simulink model "HEMS_leon"  (R2023b)
settings: Solver=FixedStepDiscrete  StartTime=0.0  StopTime=T_end  FixedStep=Ts  RelTol=1e-3  EnableMultiTasking=on
InitFcn:
  | % stepsize is now 1 per seconds cause 1 step is 1 minute
  | 
  | Ts=1/60;% 1Ts = 1minute => 60TimeSteps = 1hour
  | 
  | % Simulation Time
  | T_end = 24; % = 24 hours
StopFcn:
  | %
values from neighbouring files (symbols this model uses):
  battery_capacity = 15    [RBC.m]    (also in plot_results_HEMS.m = evalin('base', 'battery_capacity'))
  battery_efficiency = 0.95    [RBC.m]
  battery_max_charge = 5    [RBC.m]
  battery_max_soc = 90    [RBC.m]    (also in plot_results_HEMS.m = evalin('base', 'battery_max_soc'))
  battery_min_soc = 20    [RBC.m]    (also in plot_results_HEMS.m = evalin('base', 'battery_min_soc'))
  battery_soc_initial = 40    [RBC.m]
undefined symbols (not defined in the file or in its folder): A, B, battEnergy, C, D, DiscIntNeverNeededParam, optTime, x0
libraries: dspsigops x1, spspowerguiLib x1
settings Model: Creator=mas  LastModifiedBy=leons
settings SolverCC: AlgebraicLoopSolver=TrustRegion  AutoInsertRateTranBlk=on
settings DataIOCC: LimitDataPoints=on  SaveFormat=Array  SignalLoggingSaveFormat=ModelDataLogs  SaveTime=off  ReturnWorkspaceOutputs=off
settings OptimizationCC: ExpressionDepthLimit=2147483647  LifeSpan=inf
settings DebuggingCC: UnderspecifiedInitializationDetection=Classic  MergeDetectMultiDrivingBlocksExec=none  SolverPrmCheckMsg=warning  FcnCallInpInsideContextMsg=warning  UnconnectedInputMsg=warning  UnconnectedOutputMsg=warning  UnconnectedLineMsg=warning  StateNameClashWarn=warning  SFUnexpectedBacktrackingDiag=warning  SFNoUnconditionalDefaultTransitionDiag=warning  SFExecutionAtInitializationDiag=none  ArithmeticOperatorsInVariantConditions=warning
settings HardwareCC: ProdBitPerPointer=32  ProdBitPerSizeT=32  ProdBitPerPtrDiffT=32  ProdLargestAtomicFloat=None  ProdIntDivRoundTo=Undefined  ProdEndianess=Unspecified  ProdWordSize=32  ProdHWDeviceType=32-bit Generic
settings ModelReferenceCC: EnableRefExpFcnMdlSchedulingChecks=on  PropagateSignalLabelsOutOfModel=off
settings SFSimCC: SimUseLocalCustomCode=off  CustomCodeUndefinedFunction=UseInterfaceOnly
settings RTWCC: RTWUseLocalCustomCode=off  DLArmComputeVersion=19.05
settings CodeAppCC: StateflowObjectComments=on
settings GRTTargetCC: TargetLangStandard=C89/C90 (ANSI)  CombineOutputUpdateFcns=off  GRTInterface=on
settings ConfigComp: CovMetricSettings=dw  CovSaveCumulativeToWorkspaceVar=on  CovSaveSingleToWorkspaceVar=on  CovExternalEMLEnable=off  CovSFcnEnable=off

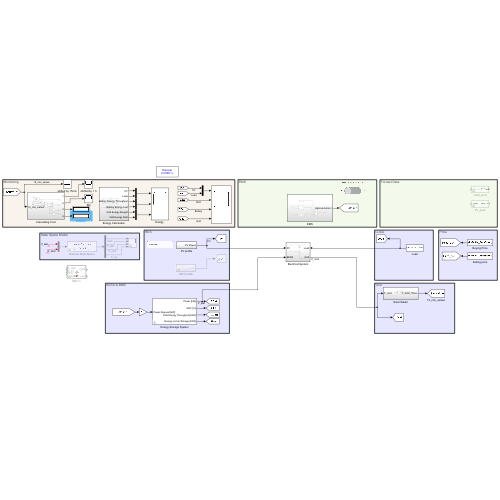
[thumbnail: Simulink's stored preview of the top-level diagram]
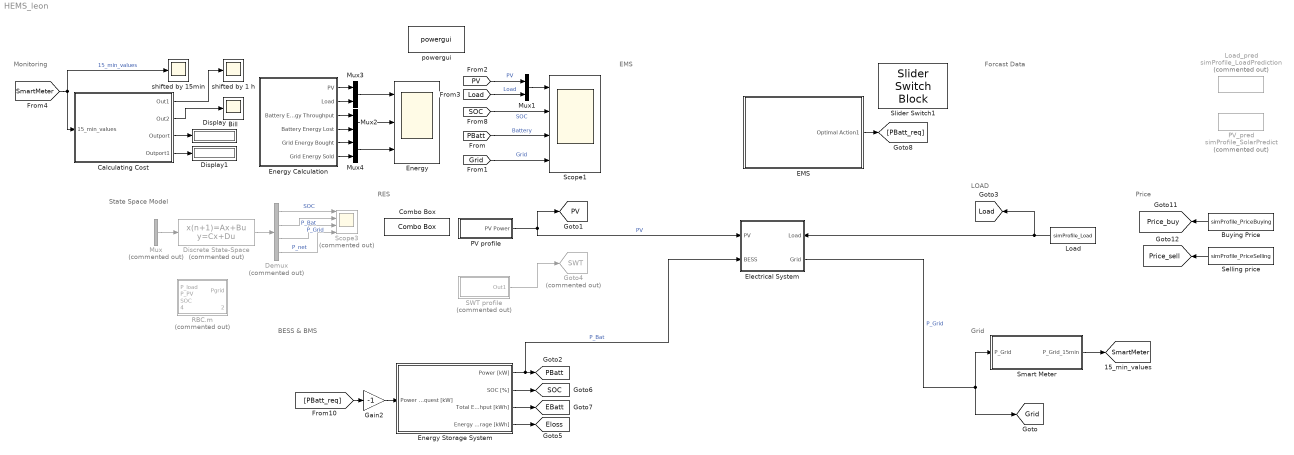
== system HEMS_leon ==
  note: State Space Model
  note: Grid
  note: BESS & BMS
  note: RES
  note: LOAD
  note: EMS
  note: Monitoring
  note: Forcast Data
  note: Price
  Bill : Scope
  Buying Price : FromWorkspace  VariableName=simProfile_PriceBuying  SampleTime=Ts*60  Interpolate=off  OutputAfterFinalValue=Holding final value
  Calculating Cost : Subsystem
  Combo Box : ComboBox  LabelPosition=Hide  SelectedLabel=Cloudy Day
      settings: Values={{'Cloudy Day', 'ClearDay'}, [1 0]}
  Demux : Demux  Commented=on
  Discrete State-Space : DiscreteStateSpace  Commented=on  A=A  B=B  C=C  D=D  InitialCondition=x0  SampleTime=-1
  Display : Display
  Display1 : Display
  EMS : Subsystem
  Electrical System : Subsystem
      settings: PortSchema="{\"entries\":[{\"content\":{\"sides\":[{\"content\":{\"connectorIds\":[\"In1\",\"Out1\"]},\"type\":\"ConnectorPlacement.EquallySpacedRectSide\",\"uuid\":\"ea2d6f6f-0b16-4ab1-9278-b701b85b7cf6\"},{\"content\":{\"connectorIds\":[\"In2\",\"In3\"],\"side\":\"RIGHT\"},\"type\":\"ConnectorPlacement.EquallySpacedRectSide\",\"uuid\":\"7f792676-012d-49e4-aa54-4a4cf568511b\"},{\"content\":{\"side\":\"TOP\"},\"type\":\"ConnectorPlacement.EquallySpacedRectSide\",\"uuid\":\"0f596cfa-1807-49b9-975a-a3b3036f9244\"}]},\"type\":\"ConnectorPlacement.EquallySpacedConnector\",\"uuid\":\"02bb58de-c0fd-4021-befc-2f3cc3c5a74e\"}],\"packageUris\":[\"http://schema.mathworks.com/mf0/Connector/R2020b\"],\"version\":\"1.0\"}"
  "Energy " : Scope  NumInputPorts=3
  Energy Calculation : Subsystem
  Energy Storage System : Subsystem  mask{Pmax=battery_max_charge, Emax=battery_capacity, SOCinit=battery_soc_initial, Eff=battery_efficiency*100, SOCmax=battery_max_soc, SOCmin=battery_min_soc}
      mask prompts: Pmax "Max Power [kW] (both for charging and discharging)"; Emax "Total Storage Energy [kWh]"; SOCinit "Initial SOC [%]"; Eff "Round Trip Efficiency [%]"; SOCmax "SOC max"; SOCmin "SOC min"
  Gain2 : Gain  Gain=-1
  Goto4 : Goto  Commented=on  GotoTag=SWT  TagVisibility=global
  Load : FromWorkspace  VariableName=simProfile_Load  SampleTime=Ts  OutputAfterFinalValue=Holding final value
  Load_pred : FromWorkspace  Commented=on  VariableName=simProfile_LoadPrediction  SampleTime=Ts  OutputAfterFinalValue=Holding final value
  Mux : Mux  Commented=on  Inputs=2
  Mux{1..4} (4 alike) : Mux  Inputs=2
  PV profile : Subsystem
  PV_pred : FromWorkspace  Commented=on  VariableName=simProfile_SolarPredict  SampleTime=Ts  OutputAfterFinalValue=Holding final value
  RBC.m : MATLAB Function  Commented=on  TreatAsAtomicUnit=on
  SWT profile : Subsystem  Commented=on
  Scope1 : Scope  NumInputPorts=4
  Scope3 : Scope  Commented=on  NumInputPorts=4
  Selling price : FromWorkspace  VariableName=simProfile_PriceSelling  SampleTime=Ts*60  Interpolate=off  OutputAfterFinalValue=Holding final value
  Slider Switch1 : SliderSwitchBlock
      settings: Values={{'RBC', 'OPT'}, [0 1]}
  Smart Meter : Subsystem
  powergui : spspowerguiLib/powergui  Priority=1  SimulationMode=Discrete  SampleTime=Ts  frequency=60  Iterations=50  frequencyindice=60  Pbase=100e6  ErrMax=1e-4  UnitsV=kV  UnitsW=MW  buscounter=0  FunctionMessages=off  echomessages=off  EnableUseOfTLC=off  CurrentSourceSwitches=off  DisableSnubberDevices=off  DisableRonSwitches=off  DisableVfSwitches=off  DisplayEquations=off  AutomaticDiscreteSolvers=off  SolverType=Tustin/Backward Euler (TBE)  Interpol=off  ExternalGateDelay=off  methode=off  Ts=100  x0status=blocks  SPID=on  SwTol=0  HookPort=off  NonlinearTolerance=1e-4  nMaxIteration=100  ContinueOnMaxIteration=off  RestoreLinks=warning  ResistiveCurrentMeasurement=off  Frange=[0:2:500]  Ylog=off  Xlog=on  ShowGrid=off  save=off  variable=ZData  structure=0  ZoomFFT=off  StartTime=0.0  cycles=1  DisplayStyle=1  fundamental=60  FreqAxis=off  MaxFrequency=1000  frequencyindicesteady=1  RmsSteady=1  display=off
  shifted by 1 h : Scope
  shifted by 15min : Scope
  tag scope: EBatt=global, Eloss=global, Grid=global, Load=global, PBatt=global, PV=global, Price_buy=global, Price_sell=global, SOC=global, SmartMeter=global
  wires:
  Energy Storage System/2(SOC [%]) -> [SOC]
  Energy Storage System/3(Total Energy Throughput [kWh]) -> [EBatt]
  PV profile/1(PV Power) -> [PV], Electrical System/2(PV)  "PV"
  Gain2/1 -> Energy Storage System/1(Power Request [kW])
  [Load] -> Mux1/2  "Load"
  [PBatt] -> Scope1/3  "Battery"
  [PV] -> Mux1/1  "PV"
  [Grid] -> Scope1/4  "Grid"
  Mux2/1 -> "Energy "/2
  Energy Storage System/4(" Energy Lost in Storage [kWh]") -> [Eloss]
  Energy Storage System/1(Power [kW]) -> Electrical System/3(BESS), [PBatt]  "P_Bat"
  Electrical System/1(Grid) -> Smart Meter/1(P_Grid), [Grid]  "P_Grid"
  Load/1 -> Electrical System/1(Load), [Load]
  ? -> Mux/2  "P_Grid"
  Demux/2 -> Scope3/2  "P_Bat"
  Demux/4 -> Scope3/4  "P_net"
  Mux/1 -> Discrete State-Space/1
  ? -> Mux/1  "P_Bat"
  Discrete State-Space/1 -> Demux/1
  Demux/1 -> Scope3/1  "SOC"
  Demux/3 -> Scope3/3  "P_Grid"
  Mux1/1 -> Scope1/1
  [SOC] -> Scope1/2  "SOC"
  Mux3/1 -> "Energy "/1
  Mux4/1 -> "Energy "/3
  EMS/1(Optimal Action1) -> [PBatt_req]
  [PBatt_req] -> Gain2/1
  Energy Calculation/1(PV) -> Mux3/1
  Energy Calculation/2(Load) -> Mux3/2
  Energy Calculation/3(Battery Energy Throughput) -> Mux2/1
  Energy Calculation/4(Battery Energy Lost) -> Mux2/2
  Energy Calculation/5(Grid Energy Bought) -> Mux4/1
  Energy Calculation/6(Grid Energy Sold) -> Mux4/2
  [SmartMeter] -> shifted by 15min/1, Calculating Cost/1(15_min_values)  "15_min_values"
  Buying Price/1 -> [Price_buy]
  Selling price/1 -> [Price_sell]
  Calculating Cost/1(Out1) -> shifted by 1 h/1
  Calculating Cost/2(Out2) -> Bill/1
  SWT profile/1(Out1) -> Goto4/1
  Smart Meter/1(P_Grid_15min) -> [SmartMeter]
  Calculating Cost/3(Outport) -> Display/1
  Calculating Cost/4(Outport1) -> Display1/1

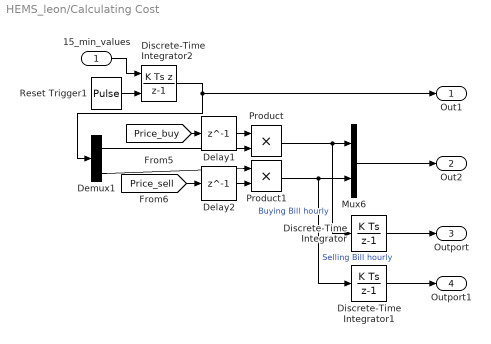
== system HEMS_leon/Calculating Cost ==
  15_min_values : Inport
  Delay1 : Delay  DelayLength=1
  Delay2 : Delay  DelayLength=1
  Demux1 : Demux  Outputs=2
  Discrete-Time Integrator : DiscreteIntegrator  SampleTime=-1  ICPrevOutput=DiscIntNeverNeededParam  ICPrevScaledInput=DiscIntNeverNeededParam
  Discrete-Time Integrator1 : DiscreteIntegrator  SampleTime=-1  ICPrevOutput=DiscIntNeverNeededParam  ICPrevScaledInput=DiscIntNeverNeededParam
  Discrete-Time Integrator2 : DiscreteIntegrator  IntegratorMethod=Integration: Backward Euler  gainval=1  ExternalReset=sampled level  SampleTime=Ts*60  ICPrevOutput=DiscIntNeverNeededParam  ICPrevScaledInput=DiscIntNeverNeededParam
  Mux6 : Mux  Inputs=2
  Product : Product
  Product1 : Product
  Reset Trigger1 : DiscretePulseGenerator  Period=60  SampleTime=Ts
  Out1 : Outport
  Out2 : Outport  Port=2
  Outport : Outport  Port=3
  Outport1 : Outport  Port=4
  wires:
  [Price_buy] -> Delay1/1
  Product1/1 -> Discrete-Time Integrator1/1, Mux6/2  "Selling Bill hourly"
  Product/1 -> Discrete-Time Integrator/1, Mux6/1  "Buying Bill hourly"
  Demux1/1 -> Product/2
  Delay2/1 -> Product1/2
  Discrete-Time Integrator2/1 -> Demux1/1, Out1/1
  [Price_sell] -> Delay2/1
  Demux1/2 -> Product1/1
  Delay1/1 -> Product/1
  Reset Trigger1/1 -> Discrete-Time Integrator2/2
  Mux6/1 -> Out2/1
  15_min_values/1 -> Discrete-Time Integrator2/1
  Discrete-Time Integrator/1 -> Outport/1
  Discrete-Time Integrator1/1 -> Outport1/1

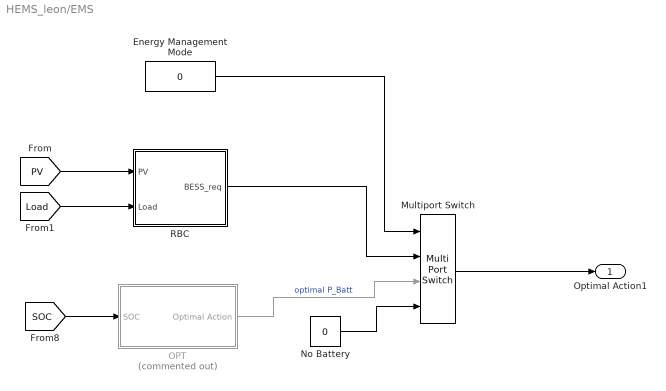
== system HEMS_leon/EMS ==
  Energy Management Mode : Constant  Value=0
  Multiport Switch : MultiPortSwitch  DataPortOrder=Zero-based contiguous  zeroidx=on  SaturateOnIntegerOverflow=off  InputSameDT=off
  No Battery : Constant  Value=0
  OPT : Subsystem  Commented=on
  RBC : Subsystem
      settings: PortSchema="{\"entries\":[{\"content\":{\"sides\":[{\"content\":{\"connectorIds\":[\"Out1\"]},\"type\":\"ConnectorPlacement.EquallySpacedRectSide\",\"uuid\":\"ea2d6f6f-0b16-4ab1-9278-b701b85b7cf6\"},{\"content\":{\"connectorIds\":[\"In1\",\"In2\"],\"side\":\"RIGHT\"},\"type\":\"ConnectorPlacement.EquallySpacedRectSide\",\"uuid\":\"7f792676-012d-49e4-aa54-4a4cf568511b\"},{\"content\":{\"side\":\"TOP\"},\"type\":\"ConnectorPlacement.EquallySpacedRectSide\",\"uuid\":\"0f596cfa-1807-49b9-975a-a3b3036f9244\"}]},\"type\":\"ConnectorPlacement.EquallySpacedConnector\",\"uuid\":\"02bb58de-c0fd-4021-befc-2f3cc3c5a74e\"}],\"packageUris\":[\"http://schema.mathworks.com/mf0/Connector/R2020b\"],\"version\":\"1.0\"}"
  Optimal Action1 : Outport  VectorParamsAs1DForOutWhenUnconnected=off
  wires:
  Multiport Switch/1 -> Optimal Action1/1
  [SOC] -> OPT/1(SOC)
  OPT/1(Optimal Action) -> Multiport Switch/3  "optimal P_Batt"
  Energy Management Mode/1 -> Multiport Switch/1
  No Battery/1 -> Multiport Switch/4
  RBC/1(BESS_req) -> Multiport Switch/2
  [PV] -> RBC/1(PV)
  [Load] -> RBC/2(Load)

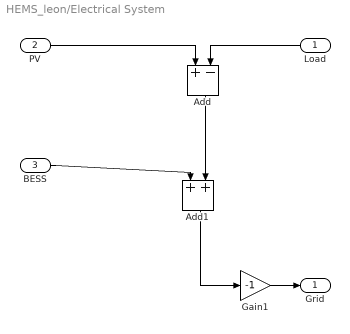
== system HEMS_leon/Electrical System ==
  Load : Inport
  PV : Inport  Port=2
  BESS : Inport  Port=3
  Add : Sum  Inputs=+-
  Add1 : Sum
  Gain1 : Gain  Gain=-1
  Grid : Outport
  wires:
  Add/1 -> Add1/2
  BESS/1 -> Add1/1
  Load/1 -> Add/2
  Add1/1 -> Gain1/1
  PV/1 -> Add/1
  Gain1/1 -> Grid/1

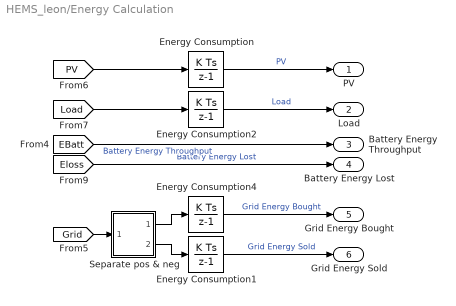
== system HEMS_leon/Energy Calculation ==
  Energy Consumption{,1..2,4} (4 alike) : DiscreteIntegrator  gainval=1  SampleTime=-1  ICPrevOutput=DiscIntNeverNeededParam  ICPrevScaledInput=DiscIntNeverNeededParam
  Separate pos & neg : Subsystem
  PV : Outport
  Load : Outport  Port=2
  Battery Energy Throughput : Outport  Port=3
  Battery Energy Lost : Outport  Port=4
  Grid Energy Bought : Outport  Port=5
  Grid Energy Sold : Outport  Port=6
  wires:
  Separate pos & neg/2(Neg) -> Energy Consumption1/1
  [Eloss] -> Battery Energy Lost/1  "Battery Energy Lost"
  [Load] -> Energy Consumption2/1
  [PV] -> Energy Consumption/1
  Separate pos & neg/1(Pos) -> Energy Consumption4/1
  Energy Consumption2/1 -> Load/1  "Load"
  Energy Consumption1/1 -> Grid Energy Sold/1  "Grid Energy Sold"
  Energy Consumption/1 -> PV/1  "PV"
  [EBatt] -> Battery Energy Throughput/1  "Battery Energy Throughput"
  Energy Consumption4/1 -> Grid Energy Bought/1  "Grid Energy Bought"
  [Grid] -> Separate pos & neg/1(Sig)

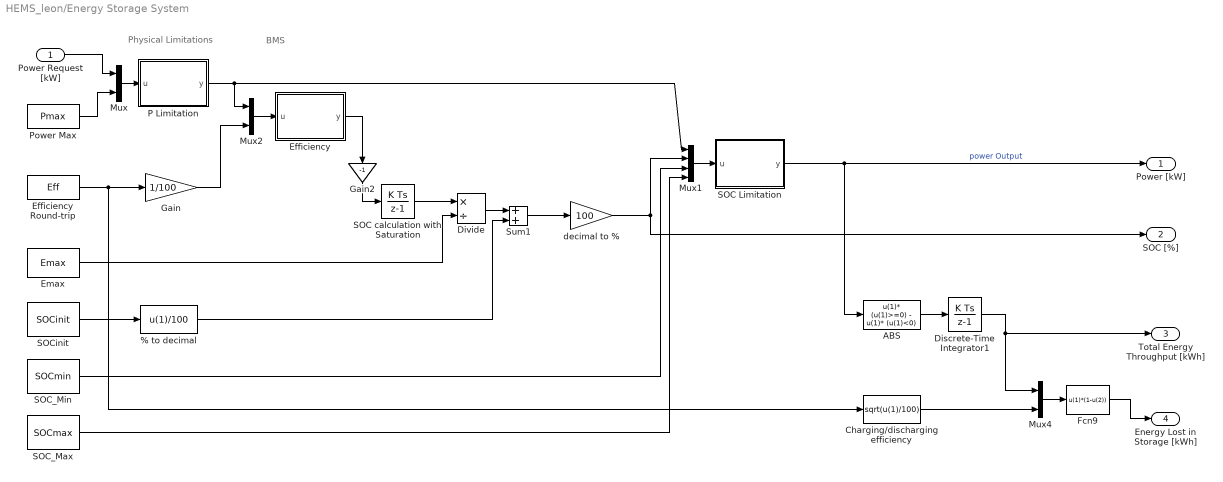
== system HEMS_leon/Energy Storage System ==
  note: Physical Limitations
  note: BMS
  Power Request [kW] : Inport
  % to decimal : Fcn  Expr=u(1)/100
  ABS : Fcn  Expr=u(1)* (u(1)>=0) - u(1)* (u(1)<0)
  Charging/discharging efficiency : Fcn  Expr=sqrt(u(1)/100)
  Discrete-Time Integrator1 : DiscreteIntegrator  gainval=1  SampleTime=-1  ICPrevOutput=DiscIntNeverNeededParam  ICPrevScaledInput=DiscIntNeverNeededParam
  Divide : Product  Inputs=*/
  Efficiency : MATLAB Function  TreatAsAtomicUnit=on
  Efficiency Round-trip : Constant  Value=Eff
  Emax : Constant  Value=Emax
  Fcn9 : Fcn  Expr=u(1)*(1-u(2))
  Gain : Gain  Gain=1/100
  Gain2 : Gain  Gain=-1
  Mux : Mux  Inputs=2
  Mux1 : Mux
  Mux2 : Mux  Inputs=2
  Mux4 : Mux  Inputs=2
  P Limitation : MATLAB Function  TreatAsAtomicUnit=on
  Power Max : Constant  Value=Pmax
  SOC Limitation : MATLAB Function  TreatAsAtomicUnit=on
  SOC calculation with Saturation : DiscreteIntegrator  gainval=1  SampleTime=-1  LimitOutput=on  UpperSaturationLimit=SOCmax/100*Emax -SOCinit/100 *Emax  LowerSaturationLimit=+SOCmin/100*Emax - SOCinit/100 *Emax  ICPrevOutput=DiscIntNeverNeededParam  ICPrevScaledInput=DiscIntNeverNeededParam
  SOC_Max : Constant  Value=SOCmax
  SOC_Min : Constant  Value=SOCmin
  SOCinit : Constant  Value=SOCinit
  Sum1 : Sum
  decimal to % : Gain  Gain=100
  Power [kW] : Outport
  SOC [%] : Outport  Port=2
  Total Energy Throughput [kWh] : Outport  Port=3
  " Energy Lost in Storage [kWh]" : Outport  Port=4
  wires:
  Mux/1 -> P Limitation/1(u)
  decimal to %/1 -> Mux1/2, SOC [%]/1
  Efficiency Round-trip/1 -> Charging/discharging efficiency/1, Gain/1
  SOCinit/1 -> % to decimal/1
  Sum1/1 -> decimal to %/1
  Divide/1 -> Sum1/1
  SOC calculation with Saturation/1 -> Divide/1
  % to decimal/1 -> Sum1/2
  Mux1/1 -> SOC Limitation/1(u)
  SOC Limitation/1(y) -> ABS/1, Power [kW]/1  "power Output"
  Gain2/1 -> SOC calculation with Saturation/1
  P Limitation/1(y) -> Mux2/1, Mux1/1
  Gain/1 -> Mux2/2
  Mux2/1 -> Efficiency/1(u)
  Discrete-Time Integrator1/1 -> Total Energy Throughput [kWh]/1, Mux4/1
  ABS/1 -> Discrete-Time Integrator1/1
  Emax/1 -> Divide/2
  Mux4/1 -> Fcn9/1
  Fcn9/1 -> " Energy Lost in Storage [kWh]"/1
  SOC_Min/1 -> Mux1/3
  SOC_Max/1 -> Mux1/4
  Power Max/1 -> Mux/2
  Power Request [kW]/1 -> Mux/1
  Charging/discharging efficiency/1 -> Mux4/2
  Efficiency/1(y) -> Gain2/1

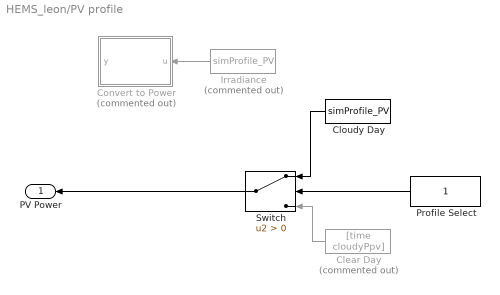
== system HEMS_leon/PV profile ==
  Clear Day : FromWorkspace  Commented=on  VariableName=[time cloudyPpv]
  Cloudy Day : FromWorkspace  VariableName=simProfile_PV
  Convert to Power : MATLAB Function  Commented=on  TreatAsAtomicUnit=on
  Irradiance : FromWorkspace  Commented=on  VariableName=simProfile_PV
  Profile Select : Constant
  Switch : Switch  Criteria=u2 > Threshold  SaturateOnIntegerOverflow=off  InputSameDT=off
  PV Power : Outport  VectorParamsAs1DForOutWhenUnconnected=off
  wires:
  Cloudy Day/1 -> Switch/1
  Profile Select/1 -> Switch/2
  Clear Day/1 -> Switch/3
  Switch/1 -> PV Power/1
  Irradiance/1 -> Convert to Power/1(u)

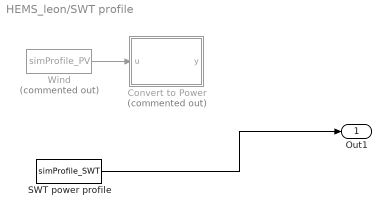
== system HEMS_leon/SWT profile ==
  Convert to Power : MATLAB Function  Commented=on  TreatAsAtomicUnit=on
  SWT power profile : FromWorkspace  VariableName=simProfile_SWT
  Wind : FromWorkspace  Commented=on  VariableName=simProfile_PV
  Out1 : Outport
  wires:
  Wind/1 -> Convert to Power/1(u)
  SWT power profile/1 -> Out1/1

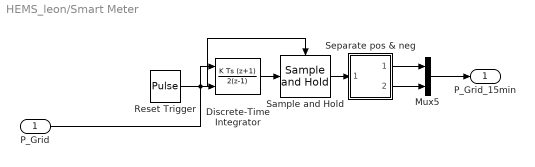
== system HEMS_leon/Smart Meter ==
  P_Grid : Inport
  Discrete-Time Integrator : DiscreteIntegrator  IntegratorMethod=Integration: Trapezoidal  gainval=1/(Ts*15)  ExternalReset=falling  SampleTime=-1  ICPrevOutput=DiscIntNeverNeededParam  ICPrevScaledInput=DiscIntNeverNeededParam
  Mux5 : Mux  Inputs=2
  Reset Trigger : DiscretePulseGenerator  Period=15  SampleTime=Ts
  Sample and Hold : dspsigops/Sample and Hold  trig=Rising edge  initCond=0  latchinput=off
  Separate pos & neg : Subsystem
  P_Grid_15min : Outport
  wires:
  Discrete-Time Integrator/1 -> Sample and Hold/1
  Sample and Hold/1 -> Separate pos & neg/1(Sig)
  Reset Trigger/1 -> Sample and Hold/Trigger, Discrete-Time Integrator/2
  Separate pos & neg/2(Neg) -> Mux5/2
  Separate pos & neg/1(Pos) -> Mux5/1
  P_Grid/1 -> Discrete-Time Integrator/1
  Mux5/1 -> P_Grid_15min/1

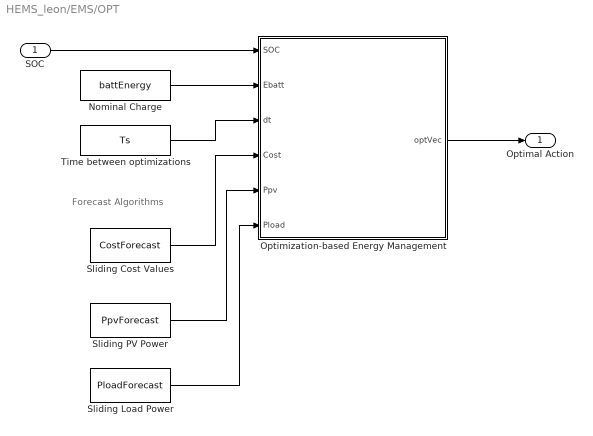
== system HEMS_leon/EMS/OPT ==
  note: Forecast Algorithms
  SOC : Inport
  Nominal Charge : Constant  Value=battEnergy
  Optimization-based Energy Management : MATLAB Function  TreatAsAtomicUnit=on  SystemSampleTime=optTime
  Sliding Cost Values : FromWorkspace  VariableName=CostForecast
  Sliding Load Power : FromWorkspace  VariableName=PloadForecast
  Sliding PV Power : FromWorkspace  VariableName=PpvForecast
  Time between optimizations : Constant  Value=Ts
  Optimal Action : Outport  VectorParamsAs1DForOutWhenUnconnected=off
  wires:
  Sliding PV Power/1 -> Optimization-based Energy Management/5(Ppv)
  Sliding Cost Values/1 -> Optimization-based Energy Management/4(Cost)
  Sliding Load Power/1 -> Optimization-based Energy Management/6(Pload)
  Nominal Charge/1 -> Optimization-based Energy Management/2(Ebatt)
  Time between optimizations/1 -> Optimization-based Energy Management/3(dt)
  SOC/1 -> Optimization-based Energy Management/1(SOC)
  Optimization-based Energy Management/1(optVec) -> Optimal Action/1

== system HEMS_leon/EMS/RBC ==
  PV : Inport
  Load : Inport  Port=2
  Add : Sum  Inputs=+-
  BESS_req : Outport
  wires:
  Load/1 -> Add/2
  PV/1 -> Add/1
  Add/1 -> BESS_req/1

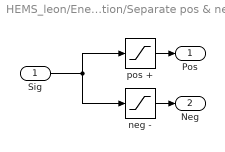
== system HEMS_leon/Energy Calculation/Separate pos & neg ==
  Sig : Inport
  neg - : Saturate  UpperLimit=0  LowerLimit=-inf
  pos + : Saturate  UpperLimit=inf  LowerLimit=0
  Pos : Outport
  Neg : Outport  Port=2
  wires:
  neg -/1 -> Neg/1
  pos +/1 -> Pos/1
  Sig/1 -> pos +/1, neg -/1

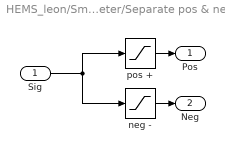
== system HEMS_leon/Smart Meter/Separate pos & neg ==
  Sig : Inport
  neg - : Saturate  UpperLimit=0  LowerLimit=-inf
  pos + : Saturate  UpperLimit=inf  LowerLimit=0
  Pos : Outport
  Neg : Outport  Port=2
  wires:
  neg -/1 -> Neg/1
  pos +/1 -> Pos/1
  Sig/1 -> pos +/1, neg -/1

== matlab function HEMS_leon/Energy Storage System/P Limitation ==
  data: u input; y output
function y = fcn(u)
y = min(max(u(1), -u(2)), u(2));

== matlab function HEMS_leon/Energy Storage System/SOC Limitation ==
  data: u input; y output
function y = fcn(u)
Pout = u(1);
SOC = u(2) ;
SOC_min = u(3);
SOC_max = u(4);

if ( SOC<=SOC_min || SOC>=SOC_max)
    Pout = 0;
end

y = Pout;

== matlab function HEMS_leon/RBC.m ==
  data: P_load input; P_PV input; SOC input; P_BESS input; Pgrid output; SOC_new output
function [Pgrid, SOC_new] = fcn(P_load, P_PV, SOC, P_BESS)
    battery_min_soc = 20

    % Net load is load minus PV generation
    net_load = P_load - P_PV;  % Net load to be supplied

    % If net load is positive, we need to either discharge the battery or buy from grid
    if net_load > 0
        if battery_soc_kWh(t) > battery_min_soc/100 *battery_capacity % If battery has charge, discharge to meet load
            discharge_power = min([battery_max_discharge, net_load, (battery_soc_kWh(t) - battery_min_soc/100 *battery_capacity)]);  % Max discharge
            battery_soc_kWh(t+1) = battery_soc_kWh(t) - discharge_power * 1/battery_efficiency;  % Update SOC
            grid_power(t) = net_load - discharge_power;  % Remaining load taken from grid
        else
            grid_power(t) = net_load;  % No battery charge left, so get all from grid
            battery_soc_kWh(t+1) = battery_soc_kWh(t);  % SOC remains unchanged
        end
    else  % If net load is negative, we have excess PV power
        excess_pv = abs(net_load);  % Excess PV available for charging or selling
        if battery_soc_kWh(t) < battery_max_soc/100 *battery_capacity  % If battery not full, charge it
            charge_power = min([battery_max_charge, excess_pv, ( battery_max_soc/100 *battery_capacity - battery_soc_kWh(t))]);  % Max charge
            battery_soc_kWh(t+1) = battery_soc_kWh(t) + charge_power * battery_efficiency;  % Update SOC
            grid_power(t) = -(excess_pv - charge_power);  % Sell remaining PV to grid
        else
            grid_power(t) = -excess_pv;  % Battery is full, sell all excess PV to grid
            battery_soc_kWh(t+1) = battery_soc_kWh(t);  % SOC remains unchanged
        end
    end

== matlab function HEMS_leon/Energy Storage System/Efficiency ==
  data: u input; y output
function y = fcn(u)
Preq = u(1);
eff = u(2) ;

if ( Preq>0) % Discharging
    y = u(1)/u(2); % for charging soc = P_bat/eff
else % charging
    y = u(1)*u(2); % for charging soc = P_bat*eff
end

== matlab function HEMS_leon/EMS/OPT/Optimization-based Energy Management ==
  data: SOC input; optVec output size=1; Ebatt input; dt input; Cost input; Ppv input; Pload input
function optVec  = fcn(SOC,Ebatt,dt,Cost,Ppv,Pload)
%#codegen

M = 241;
optVec = 0;
Pbatt = zeros(M,1);
EnergyWeight = 1;

% Energy constraints
batteryMinMax.Emax = 0.8*Ebatt;
batteryMinMax.Emin = 0.2*Ebatt;

% Power constraints
batteryMinMax.Pmin = -400e3;
batteryMinMax.Pmax = 400e3;

% Declare function (contains linprog) as extrinsic
coder.extrinsic('battSolarOptimize');

% Battery parameters
Einit = SOC/100*Ebatt;

[~,Pbatt,~] = battSolarOptimize(M,dt,Ppv,Pload,Einit,Cost,...
    EnergyWeight,batteryMinMax);

optVec = Pbatt(1);
% optVec = mean(Pbatt(1:5));

== matlab function HEMS_leon/PV profile/Convert to Power ==
  data: u input; y output
function y = fcn(u)

y = u;

== matlab function HEMS_leon/SWT profile/Convert to Power ==
  data: u input; y output
function y = fcn(u)

y = u;
